simulink model "test"  (R2021b)
settings: Solver=VariableStepAuto  StartTime=0.0  StopTime=30  RelTol=1e-3  EnableMultiTasking=on
InitFcn:
  | param
values from neighbouring files (symbols this model uses):
  P =     [P.mat]    (also in expand_path_points.m = P1 *(1 - t) + t * P2)
undefined symbols (not defined in the file or in its folder): autopilot, drawEnvironment, forces_moments, map, path_follow, path_manager, path_planner_foo, true_states
libraries: simulink x3
settings Model: Creator=beard  LastModifiedBy=hpShe
settings SolverCC: AlgebraicLoopSolver=TrustRegion
settings DataIOCC: LimitDataPoints=on  SaveFormat=Array  SignalLoggingSaveFormat=ModelDataLogs  ReturnWorkspaceOutputs=off
settings OptimizationCC: ExpressionDepthLimit=2147483647  InitFltsAndDblsToZero=on  LifeSpan=inf
settings DebuggingCC: UnderspecifiedInitializationDetection=Classic  MergeDetectMultiDrivingBlocksExec=none  SolverPrmCheckMsg=warning  FcnCallInpInsideContextMsg=warning  StateNameClashWarn=warning  SFUnexpectedBacktrackingDiag=warning  SFNoUnconditionalDefaultTransitionDiag=warning  SFExecutionAtInitializationDiag=none  SFMachineParentedDataDiag=warning  ArithmeticOperatorsInVariantConditions=warning
settings HardwareCC: ProdBitPerPointer=32  ProdBitPerSizeT=32  ProdBitPerPtrDiffT=32  ProdLargestAtomicFloat=None  ProdIntDivRoundTo=Undefined  ProdEndianess=Unspecified  ProdWordSize=32  ProdHWDeviceType=32-bit Generic
settings ModelReferenceCC: PropagateSignalLabelsOutOfModel=off
settings SFSimCC: SimUseLocalCustomCode=off  SimParseCustomCode=off  CustomCodeUndefinedFunction=UseInterfaceOnly
settings RTWCC: RTWUseLocalCustomCode=off
settings CodeAppCC: StateflowObjectComments=on
settings GRTTargetCC: TargetLangStandard=C89/C90 (ANSI)  CombineOutputUpdateFcns=off  GRTInterface=on
settings ConfigComp: CovMetricSettings=dw  CovSaveCumulativeToWorkspaceVar=on  CovSaveSingleToWorkspaceVar=on  CovExternalEMLEnable=off

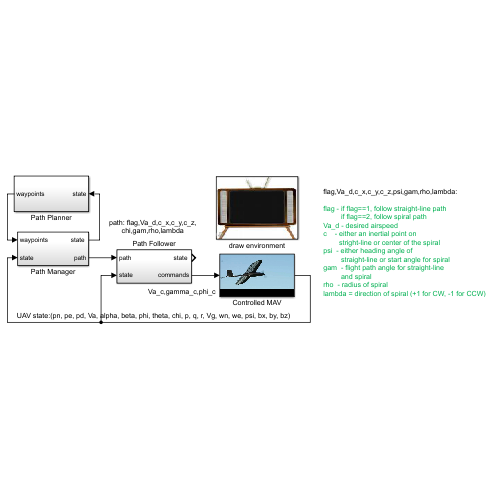
[thumbnail: Simulink's stored preview of the top-level diagram]
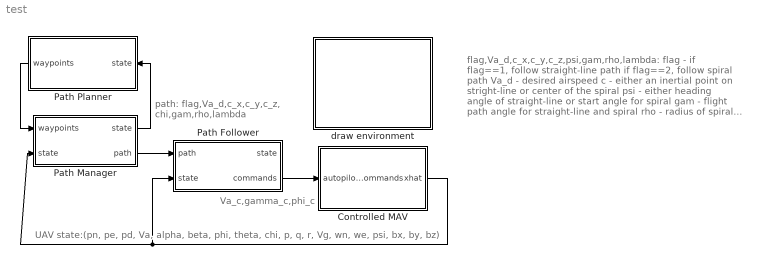
== system test ==
  note: Va_c,gamma_c,phi_c
  note: UAV state:(pn, pe, pd, Va, alpha, beta, phi, theta, chi, p, q, r, Vg, wn, we, psi, bx, by, bz)
  note: path: flag,Va_d,c_x,c_y,c_z,
      | chi,gam,rho,lambda
  note: flag,Va_d,c_x,c_y,c_z,psi,gam,rho,lambda:
      |
      | flag - if flag==1, follow straight-line path
      | if flag==2, follow spiral path
      | Va_d - desired airspeed
      | c - either an inertial point on
      | stright-line or center of the spiral
      | psi - either heading angle of
      | straight-line or start angle for spiral
      | gam - flight path angle for straight-line
      | and spiral
      | rho - radius of spiral
      | lambda = direction of spiral (+1 for CW, -1 for CCW)
  Controlled MAV : Subsystem
      mask Display: image(imread('batcam.png'))
  Path Follower : Subsystem
  Path Manager : Subsystem
  Path Planner : Subsystem
  draw environment : Subsystem  mask{map=map, R_min=P.R_min}
      mask init:
      | % parameters for drawing aircraft
      |   % scale size
      |   size = 1;
      |   fuse_l1    = 7;
      |   fuse_l2    = 4;
      |   fuse_l3    = 15;
      |   fuse_w     = 2;
      |   wing_l     = 6;
      |   wing_w     = 20;
      |   tail_l     = 3;
      |   tail_h     = 3;
      |   tailwing_w = 10;
      |   tailwing_l = 3;
      |   % colors
      |   red     = [1, 0, 0];
      |   green   = [0, 1, 0];
      |   blue    = [0, 0, 1];
      |   yellow  = [1,1,0];
      |   magenta = [0, 1, 1];
      |   
      | 
      | % define vertices and faces for aircraft
      |   V = [...
      |     fuse_l1,             0,             0;...        % point 1
      |     fuse_l2,            -fuse_w/2,     -fuse_w/2;... % point 2     
      |     fuse_l2,             fuse_w/2,     -fuse_w/2;... % point 3     
      |     fuse_l2,             fuse_w/2,      fuse_w/2;... % point 4
      |     fuse_l2,            -fuse_w/2,      fuse_w/2;... % point 5
      |    -fuse_l3,             0,             0;...        % point 6
      |     0,                   wing_w/2,      0;...        % point 7
      |    -wing_l,              wing_w/2,      0;...        % point 8
      |    -wing_l,             -wing_w/2,      0;...        % point 9
      |     0,                  -wing_w/2,      0;...        % point 10
      |    -fuse_l3+tailwing_l,  tailwing_w/2,  0;...        % point 11
      |    -fuse_l3,             tailwing_w/2,  0;...        % point 12
      |    -fuse_l3,            -tailwing_w/2,  0;...        % point 13
      |    -fuse_l3+tailwing_l, -tailwing_w/2,  0;...        % point 14
      |    -fuse_l3+tailwing_l,  0,             0;...        % point 15
      |    -fuse_l3+tailwing_l,  0,             -tail_h;...  % point 16
      |    -fuse_l3,             0,             -tail_h;...  % point 17
      |   ];
      |   
      |   F = [...
      |         1,  2,  3,  1;... % nose-top
      |         1,  3,  4,  1;... % nose-left
      |         1,  4,  5,  1;... % nose-bottom
      |         1,  5,  2,  1;... % nose-right
      |         2,  3,  6,  2;... % fuselage-top
      |         3,  6,  4,  3;... % fuselage-left
      |         4,  6,  5,  4;... % fuselage-bottom
      |         2,  5,  6,  2;... % fuselage-right
      |         7,  8,  9, 10;... % wing
      |        11, 12, 13, 14;... % tailwing
      |         6, 15, 17, 17;... % tail
      |         
      |   ];  
      |   
      |   colors = [...
      |         yellow;... % nose-top
      |         yellow;... % nose-left
      |         yellow;... % nose-bottom
      |         yellow;... % nose-right
      |         blue;... % fuselage-top
      |         blue;... % fuselage-left
      |         red;... % fuselage-bottom
      |         blue;... % fuselage-right
      |         green;... % wing
      |         green;... % tailwing
      |         blue;... % tail
      |     ];
      | 
      |   V = size*V;   % rescale vertices
      mask Display: image(imread('tv.jpg'))
  wires:
  Path Manager/2(path) -> Path Follower/1(path)
  Path Follower/2(commands) -> Controlled MAV/1(autopilot commands)
  Controlled MAV/1(xhat) -> Path Manager/2(state), Path Follower/2(state)
  Path Manager/1("state ") -> Path Planner/1(state)
  Path Planner/1(waypoints) -> Path Manager/1(waypoints)

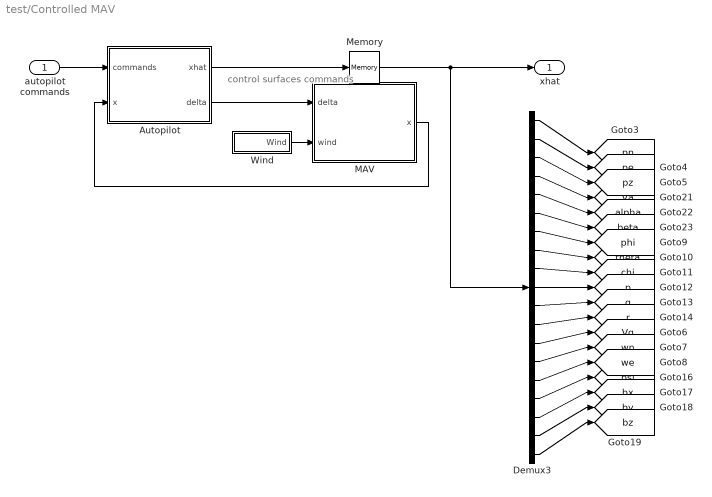
== system test/Controlled MAV ==
  note: control surfaces
      | commands
  autopilot commands : Inport
  Autopilot : Subsystem
      mask Display: image(imread('kestrel.jpg'))
  Demux3 : Demux  Outputs=19
  MAV : Subsystem
      mask Display: image(imread('batcam.png'))
  Memory : Memory
  Wind : Subsystem
  xhat : Outport
  tag scope: Va=global, Vg=global, alpha=global, beta=global, bx=global, by=global, bz=global, chi=global, p=global, pe=global, phi=global, pn=global, psi=global, pz=global, q=global, r=global, theta=global, we=global, wn=global
  wires:
  MAV/1(x) -> Autopilot/2(x)
  Autopilot/1(xhat) -> Memory/1
  autopilot commands/1 -> Autopilot/1(commands)
  Autopilot/2(delta) -> MAV/1(delta)
  Wind/1(Wind) -> MAV/2(wind)
  Demux3/16 -> [psi]
  Demux3/14 -> [wn]
  Demux3/13 -> [Vg]
  Demux3/10 -> [p]
  Demux3/15 -> [we]
  Demux3/2 -> [pe]
  Demux3/5 -> [alpha]
  Demux3/18 -> [by]
  Demux3/8 -> [theta]
  Demux3/12 -> [r]
  Demux3/1 -> [pn]
  Demux3/3 -> [pz]
  Demux3/9 -> [chi]
  Demux3/17 -> [bx]
  Memory/1 -> xhat/1, Demux3/1
  Demux3/7 -> [phi]
  Demux3/19 -> [bz]
  Demux3/4 -> [Va]
  Demux3/6 -> [beta]
  Demux3/11 -> [q]

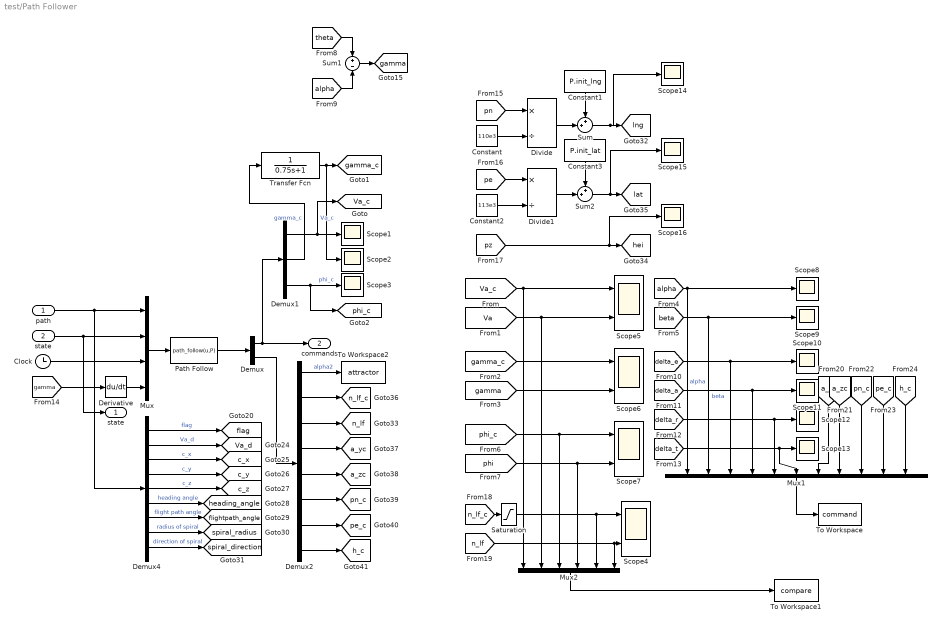
== system test/Path Follower ==
  path : Inport
  state : Inport  Port=2
  Clock : Clock
  Constant : Constant  Value=110e3
  Constant1 : Constant  Value=P.init_lng
  Constant2 : Constant  Value=113e3
  Constant3 : Constant  Value=P.init_lat
  Demux : Demux  Outputs=[3;8]
  Demux1 : Demux  Outputs=3
  Demux2 : Demux  Outputs=8
  Demux4 : Demux  Outputs=9
  Derivative : Derivative
  Divide : Product  Inputs=*/
  Divide1 : Product  Inputs=*/
  Mux : Mux
  Mux1 : Mux  Inputs=6+5
  Mux2 : Mux  Inputs=6
  Path Follow : MATLABFcn  MATLABFcn=path_follow(u,P)  OutputDimensions=3+8  SampleTime=P.Ts
  Saturation : Saturate  UpperLimit=3  LowerLimit=-1
  Scope{1..3,8..16} (12 alike) : Scope
  Scope{4..7} (4 alike) : Scope  NumInputPorts=2
  Sum : Sum  Inputs=++|
  Sum1 : Sum  Inputs=+-
  Sum2 : Sum  Inputs=++|
  To Workspace : ToWorkspace  VariableName=command  SaveFormat=Timeseries  SampleTime=-1
  To Workspace1 : ToWorkspace  VariableName=compare  SaveFormat=Timeseries  SampleTime=-1
  To Workspace2 : ToWorkspace  VariableName=attractor  SaveFormat=Timeseries  SampleTime=-1
  Transfer Fcn : TransferFcn  Denominator=[0.75 1]
  "state " : Outport
  commands : Outport  Port=2
  tag scope: Va_c=global, Va_d=global, a_yc=global, a_zc=global, c_x=global, c_y=global, c_z=global, flag=global, flightpath_angle=global, gamma=global, gamma_c=global, h_c=global, heading_angle=global, hei=global, lat=global, lng=global, n_lf=global, n_lf_c=global, pe_c=global, phi_c=global, pn_c=global, spiral_direction=global, spiral_radius=global
  wires:
  Mux/1 -> Path Follow/1
  path/1 -> Demux4/1, Mux/1
  Clock/1 -> Mux/3
  state/1 -> "state "/1, Mux/2
  Demux/1 -> Demux1/1, commands/1
  Path Follow/1 -> Demux/1
  Demux1/1 -> [Va_c], Scope1/1  "Va_c"
  Demux1/2 -> Transfer Fcn/1  "gamma_c"
  Demux1/3 -> [phi_c], Scope3/1  "phi_c"
  Demux2/1 -> To Workspace2/1  "alpha2"
  Demux/2 -> Demux2/1
  Demux2/2 -> [n_lf_c]
  Demux2/3 -> [n_lf]
  [Va_c] -> Mux2/1, Scope5/1
  [Va] -> Mux2/2, Scope5/2
  [gamma_c] -> Scope6/1
  [gamma] -> Scope6/2
  [phi_c] -> Mux2/3, Scope7/1
  [phi] -> Mux2/4, Scope7/2
  Sum1/1 -> [gamma]
  [alpha] -> Sum1/2
  [theta] -> Sum1/1
  Demux4/5 -> [c_z]  "c_z"
  Demux4/6 -> [heading_angle]  "heading angle"
  Demux4/7 -> [flightpath_angle]  "flight path angle"
  Demux4/3 -> [c_x]  "c_x"
  Demux4/4 -> [c_y]  "c_y"
  Demux4/2 -> [Va_d]  "Va_d"
  Demux4/9 -> [spiral_direction]  "direction of spiral"
  Demux4/1 -> [flag]  "flag"
  Demux4/8 -> [spiral_radius]  "radius of spiral"
  [alpha] -> Mux1/1, Scope8/1  "alpha"
  [beta] -> Mux1/2, Scope9/1  "beta"
  [delta_e] -> Scope10/1, Mux1/3
  [delta_a] -> Scope11/1, Mux1/4
  [delta_r] -> Scope12/1, Mux1/5
  [delta_t] -> Scope13/1, Mux1/6
  [gamma] -> Derivative/1
  Derivative/1 -> Mux/4
  Sum/1 -> Scope14/1, [lng]
  [pn] -> Divide/1
  Constant/1 -> Divide/2
  Divide/1 -> Sum/2
  Constant1/1 -> Sum/1
  Sum2/1 -> Scope15/1, [lat]
  Constant3/1 -> Sum2/1
  Divide1/1 -> Sum2/2
  [pe] -> Divide1/1
  Constant2/1 -> Divide1/2
  [pz] -> Scope16/1, [hei]
  [n_lf] -> Mux2/6, Scope4/2
  [n_lf_c] -> Saturation/1
  Saturation/1 -> Mux2/5, Scope4/1
  Mux1/1 -> To Workspace/1
  Mux2/1 -> To Workspace1/1
  Demux2/4 -> [a_yc]
  Demux2/5 -> [a_zc]
  Demux2/6 -> [pn_c]
  Demux2/7 -> [pe_c]
  Demux2/8 -> [h_c]
  [a_yc] -> Mux1/7
  [a_zc] -> Mux1/8
  [pn_c] -> Mux1/9
  [pe_c] -> Mux1/10
  [h_c] -> Mux1/11
  Transfer Fcn/1 -> Scope2/1, [gamma_c]

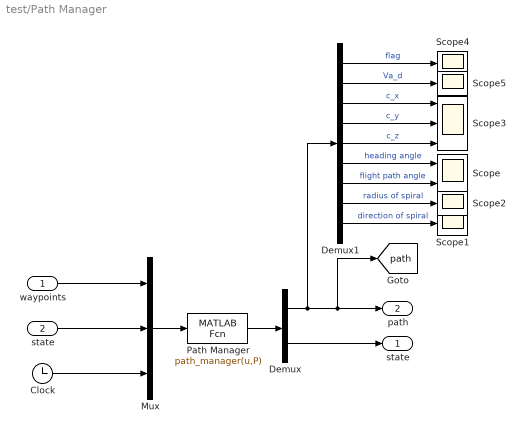
== system test/Path Manager ==
  waypoints : Inport
  state : Inport  Port=2
  Clock : Clock
  Demux : Demux  Outputs=[9;17]
  Demux1 : Demux  Outputs=9
  Mux : Mux  Inputs=3
  Path Manager : MATLABFcn  MATLABFcn=path_manager(u,P)  OutputDimensions=26  SampleTime=P.Ts
  Scope : Scope  NumInputPorts=2
  Scope{1..2,4..5} (4 alike) : Scope
  Scope3 : Scope  NumInputPorts=3
  "state " : Outport
  path : Outport  Port=2
  tag scope: path=global
  wires:
  Demux/2 -> "state "/1
  Demux/1 -> Demux1/1, path/1, [path]
  Path Manager/1 -> Demux/1
  waypoints/1 -> Mux/1
  state/1 -> Mux/2
  Clock/1 -> Mux/3
  Mux/1 -> Path Manager/1
  Demux1/1 -> Scope4/1  "flag"
  Demux1/2 -> Scope5/1  "Va_d"
  Demux1/3 -> Scope3/1  "c_x"
  Demux1/6 -> Scope/1  "heading angle"
  Demux1/7 -> Scope/2  "flight path angle"
  Demux1/9 -> Scope1/1  "direction of spiral"
  Demux1/8 -> Scope2/1  "radius of spiral"
  Demux1/4 -> Scope3/2  "c_y"
  Demux1/5 -> Scope3/3  "c_z"

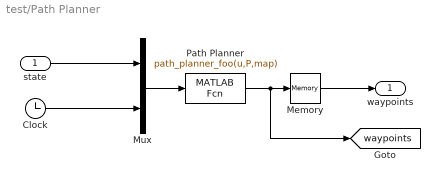
== system test/Path Planner ==
  state : Inport
  Clock : Clock
  Memory : Memory
  Mux : Mux  Inputs=2
  Path Planner : MATLABFcn  MATLABFcn=path_planner_foo(u,P,map)  OutputDimensions=1+5*P.size_waypoint_array  SampleTime=100*P.Ts
  waypoints : Outport
  tag scope: waypoints=global
  wires:
  Mux/1 -> Path Planner/1
  Clock/1 -> Mux/2
  state/1 -> Mux/1
  Path Planner/1 -> Memory/1, [waypoints]
  Memory/1 -> waypoints/1

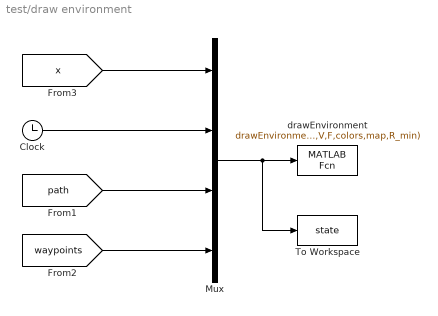
== system test/draw environment ==
  Clock : Clock
  Mux : Mux
  To Workspace : ToWorkspace  VariableName=state  SaveFormat=Timeseries  SampleTime=-1
  drawEnvironment : MATLABFcn  MATLABFcn=drawEnvironment(u,V,F,colors,map,R_min)  OutputDimensions=0  SampleTime=0.1
  wires:
  Clock/1 -> Mux/2
  [x] -> Mux/1
  Mux/1 -> To Workspace/1, drawEnvironment/1
  [path] -> Mux/3
  [waypoints] -> Mux/4

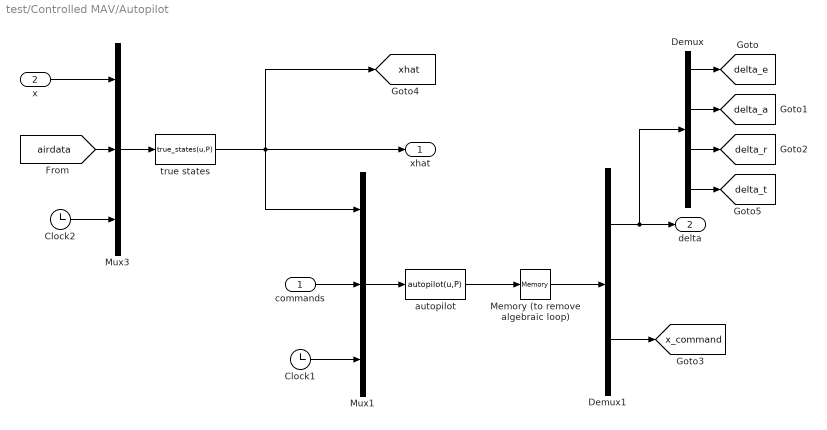
== system test/Controlled MAV/Autopilot ==
  commands : Inport
  x : Inport  Port=2
  Clock1 : Clock
  Clock2 : Clock
  Demux : Demux
  Demux1 : Demux  Outputs=[4;12]
  Memory (to remove algebraic loop) : Memory
  Mux1 : Mux  Inputs=3
  Mux3 : Mux  Inputs=3
  autopilot : MATLABFcn  MATLABFcn=autopilot(u,P)  OutputDimensions=4+12  SampleTime=P.Ts
  true states : MATLABFcn  MATLABFcn=true_states(u,P)  OutputDimensions=19  SampleTime=P.Ts
  xhat : Outport
  delta : Outport  Port=2
  tag scope: delta_a=global, delta_e=global, delta_r=global, delta_t=global, x_command=global, xhat=global
  wires:
  Memory (to remove algebraic loop)/1 -> Demux1/1
  Clock2/1 -> Mux3/3
  Clock1/1 -> Mux1/3
  x/1 -> Mux3/1
  [airdata] -> Mux3/2
  Mux3/1 -> true states/1
  true states/1 -> xhat/1, Mux1/1, [xhat]
  commands/1 -> Mux1/2
  Demux1/2 -> [x_command]
  Demux1/1 -> Demux/1, delta/1
  autopilot/1 -> Memory (to remove algebraic loop)/1
  Mux1/1 -> autopilot/1
  Demux/1 -> [delta_e]
  Demux/2 -> [delta_a]
  Demux/3 -> [delta_r]
  Demux/4 -> [delta_t]

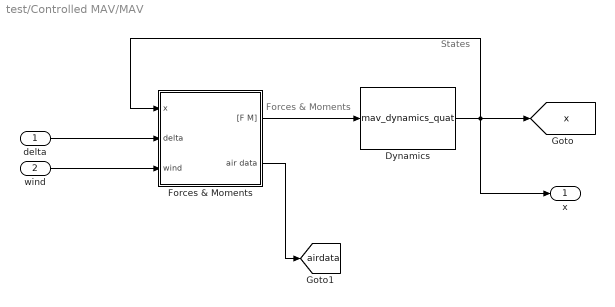
== system test/Controlled MAV/MAV ==
  note: States
  note: Forces & Moments
  delta : Inport
  wind : Inport  Port=2
  Dynamics : S-Function  FunctionName=mav_dynamics_quat  Parameters=mass,Jx,Jy,Jz,Jxz,pn0,pe0,pd0,u0,v0,w0,phi0,theta0,psi0,p0,q0,r0  SFunctionDeploymentMode=off  EnableBusSupport=off  mask{mass=P.mass, Jx=P.Jx, Jy=P.Jy, Jz=P.Jz, Jxz=P.Jxz, pn0=P.pn0, pe0=P.pe0, pd0=P.pd0, u0=P.u0, v0=P.v0, w0=P.w0, phi0=P.phi0, theta0=P.theta0, psi0=P.psi0, p0=P.p0, q0=P.q0, r0=P.r0}
      mask prompts: pn0 "Initial North position"; pe0 "Initial East position"; pd0 "Initial Down position"; u0 "Initial velocy u0"; v0 "Initial velocity v0"; w0 "Initial velocity w0"; phi0 "Initial roll angle"; theta0 "Initial pitch angle"; psi0 "Initial yaw angle"; p0 "Initial roll rate"; q0 "Initial pitch rate"; r0 "Initial yaw rate"
  Forces & Moments : Subsystem
  x : Outport
  tag scope: airdata=global, x=global
  wires:
  wind/1 -> Forces & Moments/3(wind)
  delta/1 -> Forces & Moments/2(delta)
  Forces & Moments/2(air data) -> [airdata]
  Forces & Moments/1("[F M]") -> Dynamics/1
  Dynamics/1 -> [x], Forces & Moments/1(x), x/1

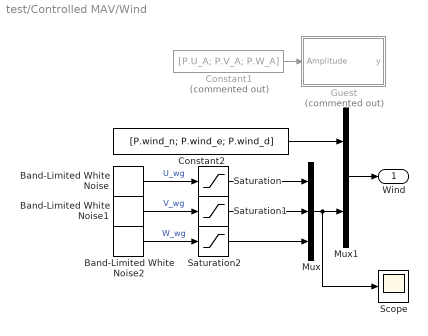
== system test/Controlled MAV/Wind ==
  Band-Limited White Noise : simulink/Sources/Band-Limited White Noise  Cov=0.1  Ts=0.1  seed=[23341]
  Band-Limited White Noise1 : simulink/Sources/Band-Limited White Noise  Cov=0.1  Ts=0.1  seed=[23341]
  Band-Limited White Noise2 : simulink/Sources/Band-Limited White Noise  Cov=0.1  Ts=0.1  seed=[23341]
  Constant1 : Constant  Commented=on  Value=[P.U_A; P.V_A; P.W_A]
  Constant2 : Constant  Value=[P.wind_n; P.wind_e; P.wind_d]
  Guest : MATLAB Function  Commented=on  TreatAsAtomicUnit=on
  Mux : Mux  Inputs=3
  Mux1 : Mux  Inputs=2
  Saturation : Saturate  UpperLimit=P.U_A  LowerLimit=-P.U_A
  Saturation1 : Saturate  UpperLimit=P.V_A  LowerLimit=-P.V_A
  Saturation2 : Saturate  UpperLimit=P.W_A  LowerLimit=-P.W_A
  Scope : Scope
  Wind : Outport
  wires:
  Mux1/1 -> Wind/1
  Constant2/1 -> Mux1/1
  Constant1/1 -> Guest/1(Amplitude)
  Mux/1 -> Scope/1, Mux1/2
  Band-Limited White Noise1/1 -> Saturation1/1  "V_wg"
  Band-Limited White Noise2/1 -> Saturation2/1  "W_wg"
  Saturation/1 -> Mux/1
  Band-Limited White Noise/1 -> Saturation/1  "U_wg"
  Saturation1/1 -> Mux/2
  Saturation2/1 -> Mux/3

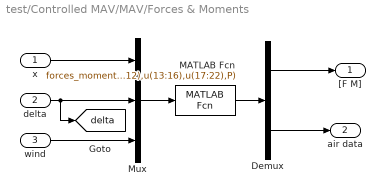
== system test/Controlled MAV/MAV/Forces & Moments ==
  x : Inport
  delta : Inport  Port=2
  wind : Inport  Port=3
  Demux : Demux  Outputs=[6;6]
  MATLAB Fcn : MATLABFcn  MATLABFcn=forces_moments(u(1:12),u(13:16),u(17:22),P)  OutputDimensions=12
  Mux : Mux  Inputs=3
  "[F M]" : Outport
  air data : Outport  Port=2
  tag scope: delta=global
  wires:
  x/1 -> Mux/1
  delta/1 -> Mux/2, [delta]
  wind/1 -> Mux/3
  MATLAB Fcn/1 -> Demux/1
  Demux/1 -> "[F M]"/1
  Mux/1 -> MATLAB Fcn/1
  Demux/2 -> air data/1

== matlab function test/Controlled MAV/Wind/Guest ==
  data: Amplitude input; y output
function y = Guest(Amplitude)
  U_A = Amplitude(1);
  V_A = Amplitude(2);
  W_A = Amplitude(3);
  
  U_wg = 2 * U_A * rand() - U_A;
  V_wg = 2 * V_A * rand() - V_A;
  W_wg = 2 * W_A * rand() - W_A;

  y = [U_wg;V_wg;W_wg];

end
